simulink model "feedback_control"  (R2024b)
settings: Solver=VariableStepAuto  StartTime=0.0  StopTime=Tend  RelTol=1e-3
values from neighbouring files (symbols this model uses):
  Ts = 0.001    [boost_data.mat]
undefined symbols (not defined in the file or in its folder): R_load
settings Model: Creator=eric  LastModifiedBy=eric

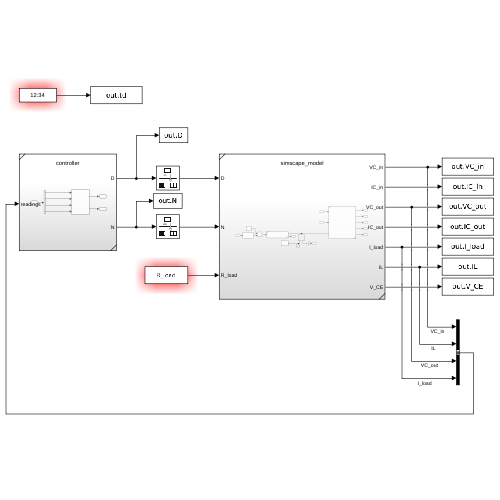
[thumbnail: Simulink's stored preview of the top-level diagram]
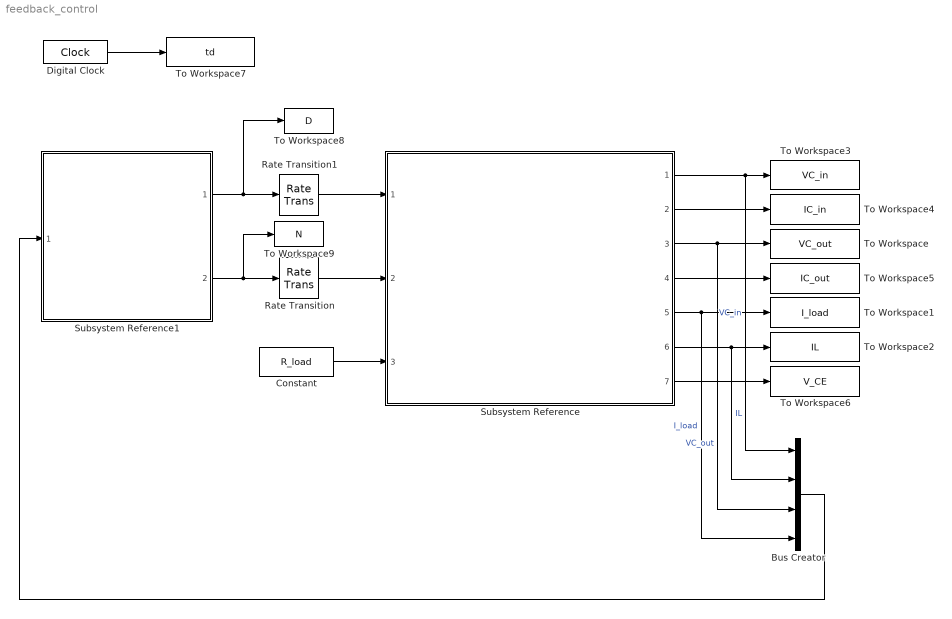
== system feedback_control ==
  Bus Creator : BusCreator  Inputs=4
  Constant : Constant  Value=R_load
  Digital Clock : DigitalClock  SampleTime=Ts
  Rate Transition : RateTransition
  Rate Transition1 : RateTransition
  Subsystem Reference : Subsystem  ReferencedSubsystem=simscape_model
  Subsystem Reference1 : Subsystem  ReferencedSubsystem=controller
  To Workspace : ToWorkspace  VariableName=VC_out  SampleTime=-1
      settings: Save2DSignal=2-D array (concatenate along first dimension)
  To Workspace1 : ToWorkspace  VariableName=I_load  SampleTime=-1
      settings: Save2DSignal=2-D array (concatenate along first dimension)
  To Workspace2 : ToWorkspace  VariableName=IL  SampleTime=-1
      settings: Save2DSignal=2-D array (concatenate along first dimension)
  To Workspace3 : ToWorkspace  VariableName=VC_in  SampleTime=-1
      settings: Save2DSignal=2-D array (concatenate along first dimension)
  To Workspace4 : ToWorkspace  VariableName=IC_in  SampleTime=-1
      settings: Save2DSignal=2-D array (concatenate along first dimension)
  To Workspace5 : ToWorkspace  VariableName=IC_out  SampleTime=-1
      settings: Save2DSignal=2-D array (concatenate along first dimension)
  To Workspace6 : ToWorkspace  VariableName=V_CE  SampleTime=-1
      settings: Save2DSignal=2-D array (concatenate along first dimension)
  To Workspace7 : ToWorkspace  VariableName=td  SampleTime=-1
      settings: Save2DSignal=2-D array (concatenate along first dimension)
  To Workspace8 : ToWorkspace  VariableName=D  SampleTime=-1
      settings: Save2DSignal=2-D array (concatenate along first dimension)
  To Workspace9 : ToWorkspace  VariableName=N  SampleTime=-1
      settings: Save2DSignal=2-D array (concatenate along first dimension)
  wires:
  Subsystem Reference1/1 -> To Workspace8/1, Rate Transition1/1
  Subsystem Reference1/2 -> To Workspace9/1, Rate Transition/1
  Constant/1 -> Subsystem Reference/3
  Subsystem Reference/3 -> Bus Creator/3, To Workspace/1  "VC_out"
  Subsystem Reference/5 -> Bus Creator/4, To Workspace1/1  "I_load"
  Subsystem Reference/6 -> Bus Creator/2, To Workspace2/1  "IL"
  Subsystem Reference/1 -> Bus Creator/1, To Workspace3/1  "VC_in"
  Subsystem Reference/2 -> To Workspace4/1
  Subsystem Reference/4 -> To Workspace5/1
  Subsystem Reference/7 -> To Workspace6/1
  Rate Transition1/1 -> Subsystem Reference/1
  Rate Transition/1 -> Subsystem Reference/2
  Digital Clock/1 -> To Workspace7/1
  Bus Creator/1 -> Subsystem Reference1/1
